simulink model "test_NN"  (R2025a)
settings: Solver=FixedStepAuto  StartTime=0.0  StopTime=10.0  FixedStep=0.001  RelTol=1e-3
undefined symbols (not defined in the file or in its folder): torch
libraries: deeplib x2, pycoexlib x1
settings Model: SimulationMode=accelerator  Creator=Asus  LastModifiedBy=Asus

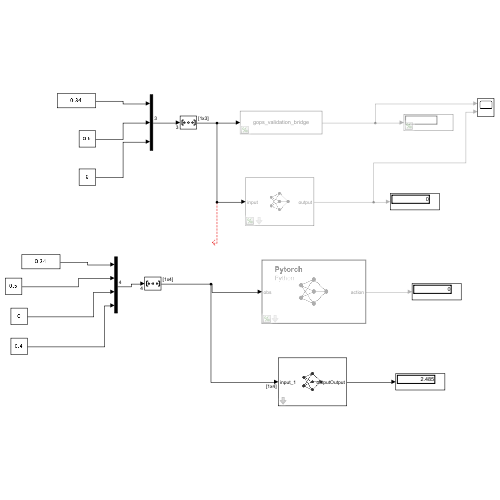
[thumbnail: Simulink's stored preview of the top-level diagram]
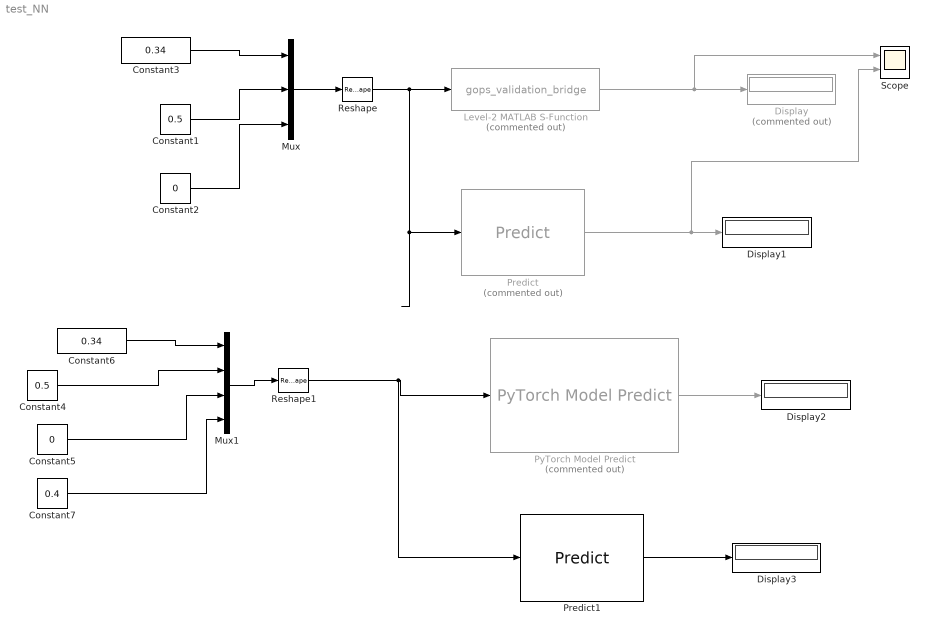
== system test_NN ==
  Constant1 : Constant  Value=0.5
  Constant2 : Constant  Value=0
  Constant3 : Constant  Value=0.34
  Constant4 : Constant  Value=0.5
  Constant5 : Constant  Value=0
  Constant6 : Constant  Value=0.34
  Constant7 : Constant  Value=0.4
  Display : Display  Commented=on
  Display1 : Display
  Display2 : Display
  Display3 : Display
  Level-2 MATLAB S-Function : M-S-Function  Commented=on  FunctionName=gops_validation_bridge  Parameters='NN_controller_PPO.pt'
  Mux : Mux  Inputs=3
  Mux1 : Mux
  Predict : deeplib/Predict  Commented=on  Network=Network from MAT-file  NetworkFunction=squeezenet  NetworkFilePath=D:\Project\SynologyDrive\Imp_fcn_cal\RL_model\onnx_model.mat  MiniBatchSize=128  InputDataFormats={ 'input_1', 'UU' }  Predictions=on  Activations={}  ForceInterpretedSim=off  EnableDLNetwork=on  LastKnownNetworkFilePath='D:\Project\SynologyDrive\Imp_fcn_cal\RL_model\onnx_model.mat'  LastKnownNetworkTimeStamp=739855.706932870321907103061676025390625
  Predict1 : deeplib/Predict  Network=Network from MAT-file  NetworkFunction=squeezenet  NetworkFilePath=D:\Project\GOPS\mdl\RL_model\TD3_46071_opt.mat  MiniBatchSize=128  InputDataFormats={ 'input_1', 'UU' }  Predictions=on  Activations={}  ForceInterpretedSim=off  EnableDLNetwork=on  LastKnownNetworkFilePath='D:\Project\GOPS\mdl\RL_model\TD3_46071_opt.mat'  LastKnownNetworkTimeStamp=739967.670486111077480018138885498046875
  PyTorch Model Predict : pycoexlib/PyTorch Model Predict  Commented=on  ModelFile=D:\Project\GOPS\mdl\RL_model\td3_46071_opt.pt  LoadCommandPopup=torch.jit.load()  DeviceComboBox=cpu  InputTable={ 'obs', 'float32', '', '[2]' }  OutputTable={ 'action', '', '' }  SampleTime=0.01  TorchLoadCommand=torch.jit.load()  Device=cpu  InputDatatypes=float32  InputNumDims=[2]  InputPermutations=[]  OutputPermutations=[]  PythonCoexecutionBlockType=PyTorchModelBlock  VariableOutputMaxSizes=[]
  Reshape : Reshape  OutputDimensionality=Row vector (2-D)
  Reshape1 : Reshape  OutputDimensionality=Row vector (2-D)
  Scope : Scope  NumInputPorts=2
      settings: ActiveDisplayYMinimum=-0.14687764830887318  ActiveDisplayYMaximum=0.016319738700985905
  wires:
  Constant3/1 -> Mux/1
  Constant1/1 -> Mux/2
  Constant2/1 -> Mux/3
  Mux/1 -> Reshape/1
  Level-2 MATLAB S-Function/1 -> Scope/1, Display/1
  Reshape/1 -> Predict/1, Level-2 MATLAB S-Function/1
  Predict/1 -> Scope/2, Display1/1
  PyTorch Model Predict/1 -> Display2/1
  Mux1/1 -> Reshape1/1
  Constant5/1 -> Mux1/3
  Constant4/1 -> Mux1/2
  Constant6/1 -> Mux1/1
  Reshape1/1 -> Predict1/1, PyTorch Model Predict/1
  Constant7/1 -> Mux1/4
  Predict1/1 -> Display3/1
